simulink model "basic_traffic_signal_2019v"  (R2019b)
settings: Solver=VariableStepAuto  StartTime=0.0  StopTime=inf  RelTol=1e-3
settings Model: Creator=Brigosha_Guest  LastModifiedBy=Brigosha_Guest
settings DebuggingCC: UnconnectedInputMsg=none  UnconnectedOutputMsg=none  UnconnectedLineMsg=none  SFMachineParentedDataDiag=error
settings ModelReferenceCC: EnableRefExpFcnMdlSchedulingChecks=off
settings RTWCC: Description=Generic Real-Time Target

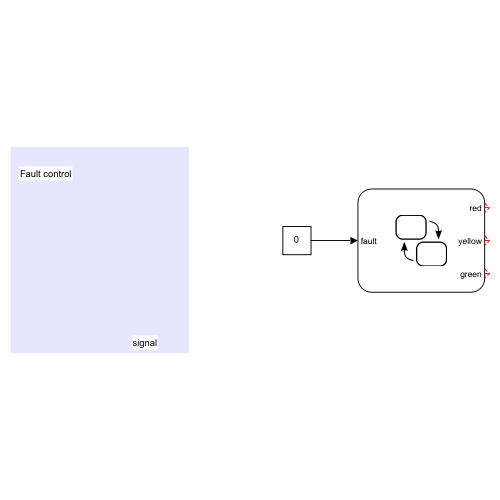
[thumbnail: Simulink's stored preview of the top-level diagram]
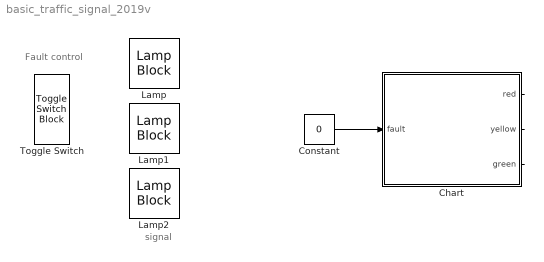
== system basic_traffic_signal_2019v ==
  note: signal
  note: Fault control
  Chart : Stateflow chart  TreatAsAtomicUnit=on
  Constant : Constant  Value=0
  Lamp : LampBlock  LabelPosition=Hide
  Lamp1 : LampBlock  LabelPosition=Hide
  Lamp2 : LampBlock  LabelPosition=Hide
  Toggle Switch : ToggleSwitchBlock  LabelPosition=Hide
      settings: Values={{'Off', 'On'}, [0 1]}
  wires:
  Constant/1 -> Chart/1(fault)
  Chart/3(green) -> ?
  Chart/1(red) -> ?
  Chart/2(yellow) -> ?

== stateflow chart basic_traffic_signal_2019v/Chart ==
  state NormalMode
    state Stop
      entry:
      red=1;
      yellow=0;
      green=0;
    state PrepareToStop
      entry:
      red=0;
      yellow=1;
      green=0;
    state Go
      entry:
      red=0;
      yellow=0;
      green=1;
    (default) -> Stop
    Stop -> PrepareToStop : after(3,sec)
    PrepareToStop -> Go : after(4,sec)
    Go -> Stop : after(10,sec)
  state FaultMode
    entry:
    yellow=0;
    green=0;
    state BlinkOff
      entry:
      red=0;
    state BlinkOn
      entry:
      red=1;
    (default) -> BlinkOff
    BlinkOff -> BlinkOn : after(2,sec)
    BlinkOn -> BlinkOff : after(2,sec)
  (default) -> NormalMode
  NormalMode -> FaultMode : [fault==1]
  FaultMode -> NormalMode : [fault==0]
  data: red output; yellow output; green output; fault input
